simulink model "etrobocon_host"  (R2013b)
settings: Solver=FixedStepDiscrete  StartTime=0.0  StopTime=inf  FixedStep=Ts  RelTol=1e-3
PreLoadFcn:
  | %addpath('C:\Users\ming\Desktop\LEGO_NXT\ETRoboCon2013\data_types\enumerations');
  | Ts = 0.1;
undefined symbols (not defined in the file or in its folder): Green, led0, Stateflow
libraries: embdlinuxlib x11, simulink x6, aerolibanimutils x1
CloseFcn:
  | rmpath('C:\Users\ming\Desktop\LEGO_NXT\ETRoboCon2013\data_types\enumerations');
settings Model: ExtModeTrigDuration=100  Creator=scastro  LastModifiedBy=ming
settings OptimizationCC: OptimizeModelRefInitCode=on  LifeSpan=Inf
settings DebuggingCC: SolverPrmCheckMsg=none
settings HardwareCC: ProdLargestAtomicInteger=Long  ProdLargestAtomicFloat=Double  ProdEndianess=LittleEndian  ProdHWDeviceType=ARM Compatible->ARM Cortex
settings RTWCC: SystemTargetFile=realtime.tlc  GenerateMakefile=off  TemplateMakefile=realtime.tmf  Description=Run on Target Hardware  RTWVerbose=off  ProcessScript=realtime_make_rtw_hook
settings STFCustomTargetCC: TargetLibSuffix=.a  GenerateSampleERTMain=on  ERTCustomFileBanners=on  SupportNonInlinedSFcns=off  SupportVariableSizeSignals=on  MATLABClassNameForMDSCustomization=Simulink.SoftwareTarget.ERTCustomization  GRTInterface=off  SystemTargetFile=realtime.tlc
settings ERTTargetCC: CodeReplacementLibrary=ANSI_C  GenerateSampleERTMain=on  ParMdlRefBuildCompliant=off  CompOptLevelCompliant=off  ConcurrentExecutionCompliant=off  CombineOutputUpdateFcns=off  ERTFirstTimeCompliant=off  SupportContinuousTime=on  SupportVariableSizeSignals=on  ModelStepFunctionPrototypeControlCompliant=off  CPPClassGenCompliant=off  ExtModeMexArgs='192.168.2.6' 0 17725  InlinedParameterPlacement=NonHierarchical  ERTSrcFileBannerTemplate=realtime_code_template.cgt  ERTHdrFileBannerTemplate=realtime_code_template.cgt  ERTDataSrcFileTemplate=realtime_code_template.cgt  ERTDataHdrFileTemplate=realtime_code_template.cgt  ERTCustomFileTemplate=realtime_file_process.tlc

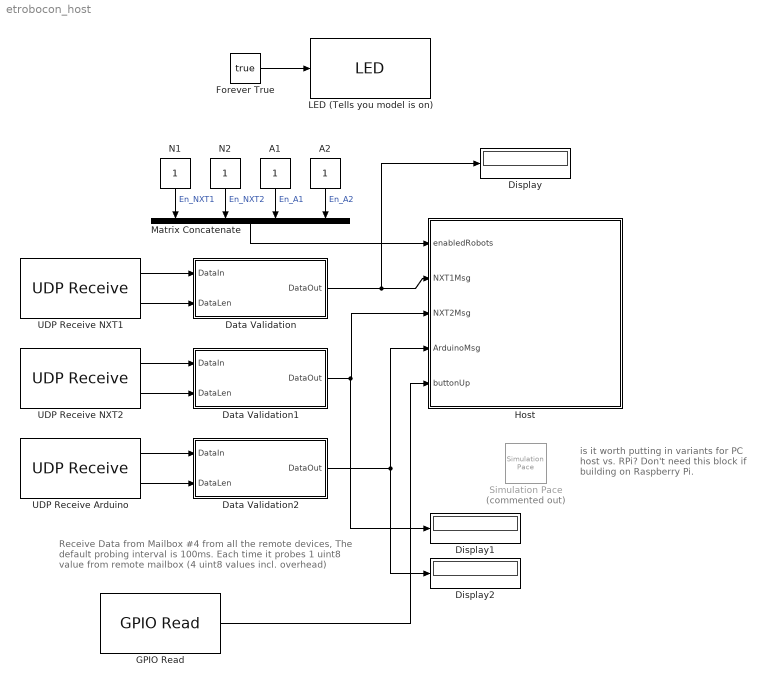
== system etrobocon_host ==
  note: is it worth putting in variants for
      | PC host vs. RPi?
      |
      | Don't need this block if building on
      | Raspberry Pi.
  note: Receive Data from Mailbox #4 from all the remote devices,
      | The default probing interval is 100ms. Each time it probes 1
      | uint8 value from remote mailbox (4 uint8 values incl. overhead)
  A1 : Constant
  A2 : Constant
  Data Validation : Subsystem
  Data Validation1 : Subsystem
  Data Validation2 : Subsystem
  Display : Display
  Display1 : Display
  Display2 : Display
  Forever True : Constant  Value=true  OutDataTypeStr=boolean
  GPIO Read : embdlinuxlib/GPIO Read  board=Model B Rev2  gpio=4  internalResistor=Off  sampleTime=Ts  direction=Input  blockPlatform=Raspberry Pi
  Host : Stateflow chart  TreatAsAtomicUnit=on
  LED (Tells you model is on) : embdlinuxlib/LED  board=Model B Rev2  led=led0 (Green)  blockPlatform=Raspberry Pi
  Matrix Concatenate : Concatenate  NumInputs=4  ConcatenateDimension=2
  N1 : Constant
  N2 : Constant
  Simulation Pace : aerolibanimutils/Simulation Pace  Commented=on  SimulationPace=1  SleepMode=MATLAB Thread  OutputPaceError=off  SampleTime=-1
      settings: AttributesFormatString=%<SimulationPace> sec/sec
  UDP Receive Arduino : embdlinuxlib/UDP Receive  localURL='0.0.0.0'  localPort=35715  remoteURL='0.0.0.0'  remotePort=-1  recvBufferSize=8192  signalDatatype=uint8  dims=4  isVarSize=off  showBlockingTime=off  blockingTime=0  sampletime=Ts  blockPlatform=Raspberry Pi
  "UDP Receive NXT1 " : embdlinuxlib/UDP Receive  localURL='0.0.0.0'  localPort=35713  remoteURL='0.0.0.0'  remotePort=-1  recvBufferSize=8192  signalDatatype=uint8  dims=4  isVarSize=off  showBlockingTime=off  blockingTime=0  sampletime=Ts  blockPlatform=Raspberry Pi
  UDP Receive NXT2 : embdlinuxlib/UDP Receive  localURL='0.0.0.0'  localPort=35714  remoteURL='0.0.0.0'  remotePort=-1  recvBufferSize=8192  signalDatatype=uint8  dims=4  isVarSize=off  showBlockingTime=off  blockingTime=0  sampletime=Ts  blockPlatform=Raspberry Pi
  wires:
  Data Validation/1(DataOut) -> Display/1, Host/2(NXT1Msg)
  N1/1 -> Matrix Concatenate/1  "En_NXT1"
  N2/1 -> Matrix Concatenate/2  "En_NXT2"
  A1/1 -> Matrix Concatenate/3  "En_A1"
  A2/1 -> Matrix Concatenate/4  "En_A2"
  Matrix Concatenate/1 -> Host/1(enabledRobots)
  UDP Receive Arduino/1 -> Data Validation2/1(DataIn)
  UDP Receive Arduino/2 -> Data Validation2/2(DataLen)
  "UDP Receive NXT1 "/2 -> Data Validation/2(DataLen)
  "UDP Receive NXT1 "/1 -> Data Validation/1(DataIn)
  UDP Receive NXT2/2 -> Data Validation1/2(DataLen)
  UDP Receive NXT2/1 -> Data Validation1/1(DataIn)
  Data Validation1/1(DataOut) -> Display1/1, Host/3(NXT2Msg)
  Data Validation2/1(DataOut) -> Host/4(ArduinoMsg), Display2/1
  GPIO Read/1 -> Host/5(buttonUp)
  Forever True/1 -> LED (Tells you model is on)/1

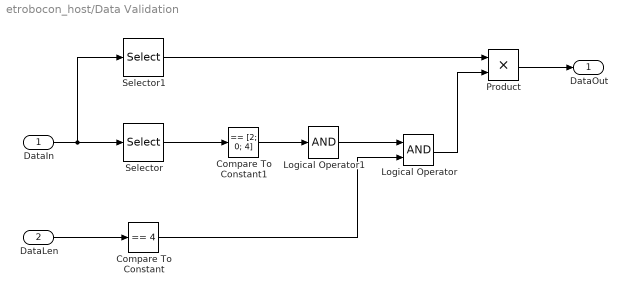
== system etrobocon_host/Data Validation ==
  DataIn : Inport
  DataLen : Inport  Port=2
  Compare To Constant : simulink/Logic and Bit Operations/Compare To Constant  relop===  const=4  OutDataTypeStr=boolean
  Compare To Constant1 : simulink/Logic and Bit Operations/Compare To Constant  relop===  const=[2; 0; 4]  OutDataTypeStr=boolean
  Logical Operator : Logic  AllPortsSameDT=off  OutDataTypeStr=boolean
  Logical Operator1 : Logic  Inputs=1  AllPortsSameDT=off  OutDataTypeStr=boolean
  Product : Product  OutDataTypeStr=uint8
  Selector : Selector  InputPortWidth=4  IndexOptions=Index vector (dialog)  Indices=[1 2 3]  OutputSizes=1
  Selector1 : Selector  InputPortWidth=4  IndexOptions=Index vector (dialog)  Indices=[4]  OutputSizes=1
  DataOut : Outport
  wires:
  Logical Operator/1 -> Product/2
  Compare To Constant/1 -> Logical Operator/2
  Logical Operator1/1 -> Logical Operator/1
  DataIn/1 -> Selector1/1, Selector/1
  DataLen/1 -> Compare To Constant/1
  Selector/1 -> Compare To Constant1/1
  Compare To Constant1/1 -> Logical Operator1/1
  Selector1/1 -> Product/1
  Product/1 -> DataOut/1

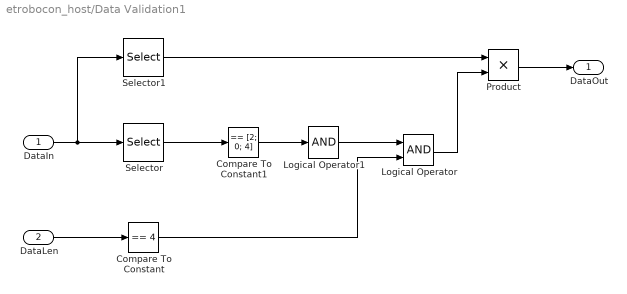
== system etrobocon_host/Data Validation1 ==
  DataIn : Inport
  DataLen : Inport  Port=2
  Compare To Constant : simulink/Logic and Bit Operations/Compare To Constant  relop===  const=4  OutDataTypeStr=boolean
  Compare To Constant1 : simulink/Logic and Bit Operations/Compare To Constant  relop===  const=[2; 0; 4]  OutDataTypeStr=boolean
  Logical Operator : Logic  AllPortsSameDT=off  OutDataTypeStr=boolean
  Logical Operator1 : Logic  Inputs=1  AllPortsSameDT=off  OutDataTypeStr=boolean
  Product : Product  OutDataTypeStr=uint8
  Selector : Selector  InputPortWidth=4  IndexOptions=Index vector (dialog)  Indices=[1 2 3]  OutputSizes=1
  Selector1 : Selector  InputPortWidth=4  IndexOptions=Index vector (dialog)  Indices=[4]  OutputSizes=1
  DataOut : Outport
  wires:
  Product/1 -> DataOut/1
  Selector1/1 -> Product/1
  Compare To Constant1/1 -> Logical Operator1/1
  Selector/1 -> Compare To Constant1/1
  DataLen/1 -> Compare To Constant/1
  DataIn/1 -> Selector/1, Selector1/1
  Logical Operator1/1 -> Logical Operator/1
  Compare To Constant/1 -> Logical Operator/2
  Logical Operator/1 -> Product/2

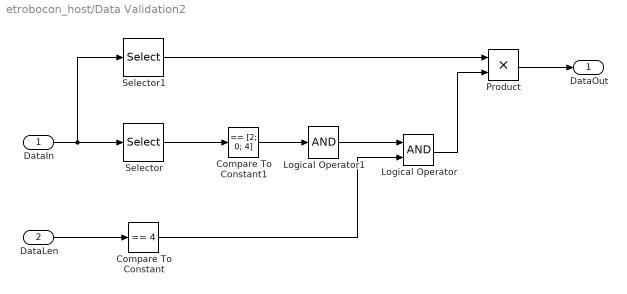
== system etrobocon_host/Data Validation2 ==
  DataIn : Inport
  DataLen : Inport  Port=2
  Compare To Constant : simulink/Logic and Bit Operations/Compare To Constant  relop===  const=4  OutDataTypeStr=boolean
  Compare To Constant1 : simulink/Logic and Bit Operations/Compare To Constant  relop===  const=[2; 0; 4]  OutDataTypeStr=boolean
  Logical Operator : Logic  AllPortsSameDT=off  OutDataTypeStr=boolean
  Logical Operator1 : Logic  Inputs=1  AllPortsSameDT=off  OutDataTypeStr=boolean
  Product : Product  OutDataTypeStr=uint8
  Selector : Selector  InputPortWidth=4  IndexOptions=Index vector (dialog)  Indices=[1 2 3]  OutputSizes=1
  Selector1 : Selector  InputPortWidth=4  IndexOptions=Index vector (dialog)  Indices=[4]  OutputSizes=1
  DataOut : Outport
  wires:
  Logical Operator/1 -> Product/2
  Compare To Constant/1 -> Logical Operator/2
  Logical Operator1/1 -> Logical Operator/1
  DataIn/1 -> Selector1/1, Selector/1
  DataLen/1 -> Compare To Constant/1
  Selector/1 -> Compare To Constant1/1
  Compare To Constant1/1 -> Logical Operator1/1
  Selector1/1 -> Product/1
  Product/1 -> DataOut/1

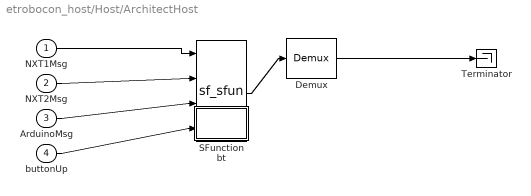
== system etrobocon_host/Host/ArchitectHost ==
  NXT1Msg : Inport
  NXT2Msg : Inport  Port=2
  ArduinoMsg : Inport  Port=3
  buttonUp : Inport  Port=4
  " Demux " : Demux  Outputs=1
  " SFunction " : S-Function  Tag=Stateflow S-Function etrobocon_host 5  FunctionName=sf_sfun  PortCounts=[4 1]  EnableBusSupport=off
  " Terminator " : Terminator
  bt : Stateflow chart  TreatAsAtomicUnit=on
  wires:
  NXT1Msg/1 -> " SFunction "/1
  NXT2Msg/1 -> " SFunction "/2
  ArduinoMsg/1 -> " SFunction "/3
  buttonUp/1 -> " SFunction "/4
  " Demux "/1 -> " Terminator "/1
  " SFunction "/1 -> " Demux "/1

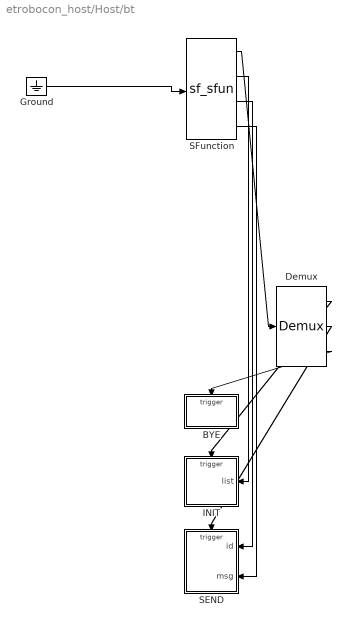
== system etrobocon_host/Host/bt ==
  " Demux " : Demux  Outputs=3
  " Ground " : Ground
  " SFunction " : S-Function  Tag=Stateflow S-Function etrobocon_host 2  FunctionName=sf_sfun  PortCounts=[1 4]  EnableBusSupport=off
  BYE : Subsystem
      settings: UndoDeleteFcn=Stateflow.SLINSF.SimulinkMan.restorePreDeleteFcn  PreDeleteFcn=Stateflow.SLINSF.SimulinkMan.removePreDeleteFcn
  INIT : Subsystem
      settings: UndoDeleteFcn=Stateflow.SLINSF.SimulinkMan.restorePreDeleteFcn  PreDeleteFcn=Stateflow.SLINSF.SimulinkMan.removePreDeleteFcn
  SEND : Subsystem
      settings: UndoDeleteFcn=Stateflow.SLINSF.SimulinkMan.restorePreDeleteFcn  PreDeleteFcn=Stateflow.SLINSF.SimulinkMan.removePreDeleteFcn
  wires:
  " SFunction "/2 -> INIT/1(list)
  " Demux "/1 -> INIT/Trigger
  " SFunction "/3 -> SEND/1(id)
  " SFunction "/4 -> SEND/2(msg)
  " Demux "/2 -> SEND/Trigger
  " Demux "/3 -> BYE/Trigger
  " Ground "/1 -> " SFunction "/1
  " SFunction "/1 -> " Demux "/1

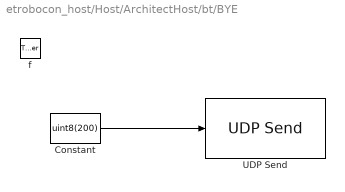
== system etrobocon_host/Host/ArchitectHost/bt/BYE ==
  f : TriggerPort  TriggerType=function-call
      settings: CopyFcn=Stateflow.SLINSF.SimulinkMan.removeBlockPreDeleteFcn  PreDeleteFcn=Stateflow.SLINSF.SimulinkMan.unsafePredeleteFcn
  Constant : Constant  Value=uint8(200)  VectorParams1D=off
      settings: SamplingMode=Frame based
  UDP Send : embdlinuxlib/UDP Send  remoteURL='127.0.0.1'  remotePort=35712  localURL='255.255.255.255'  localPortSource=Automatically determine  localPort=-1  sampletime=-1  blockPlatform=Raspberry Pi  separateLengthPort=0
  wires:
  Constant/1 -> UDP Send/1

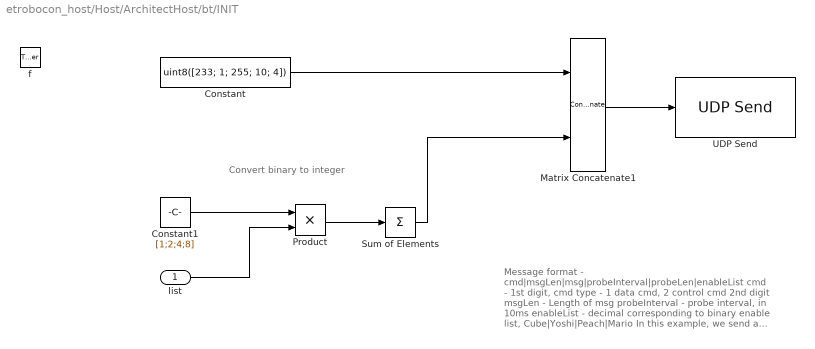
== system etrobocon_host/Host/ArchitectHost/bt/INIT ==
  note: Message format -
      | cmd|msgLen|msg|probeInterval|probeLen|enableList
      | cmd - 1st digit, cmd type - 1 data cmd, 2 control cmd
      | 2nd digit
      | msgLen - Length of msg
      | probeInterval - probe interval, in 10ms
      | enableList - decimal corresponding to binary enable list,
      | Cube|Yoshi|Peach|Mario
      | In this example, we send a unint8 255
  note: Convert binary to integer
  list : Inport  OutDataTypeStr=double  PortDimensions=4
  f : TriggerPort  TriggerType=function-call
      settings: CopyFcn=Stateflow.SLINSF.SimulinkMan.removeBlockPreDeleteFcn  PreDeleteFcn=Stateflow.SLINSF.SimulinkMan.unsafePredeleteFcn
  Constant : Constant  Value=uint8([233; 1; 255; 10; 4])  VectorParams1D=off
      settings: SamplingMode=Frame based
  Constant1 : Constant  Value=[1;2;4;8]
  Matrix Concatenate1 : Concatenate  Mode=Multidimensional array
  Product : Product
  Sum of Elements : Sum  Inputs=+  AccumDataTypeStr=uint8  OutDataTypeStr=uint8
  UDP Send : embdlinuxlib/UDP Send  remoteURL='127.0.0.1'  remotePort=35712  localURL='255.255.255.255'  localPortSource=Automatically determine  localPort=-1  sampletime=-1  blockPlatform=Raspberry Pi  separateLengthPort=0
  wires:
  Sum of Elements/1 -> Matrix Concatenate1/2
  Constant/1 -> Matrix Concatenate1/1
  Matrix Concatenate1/1 -> UDP Send/1
  Product/1 -> Sum of Elements/1
  Constant1/1 -> Product/1
  list/1 -> Product/2

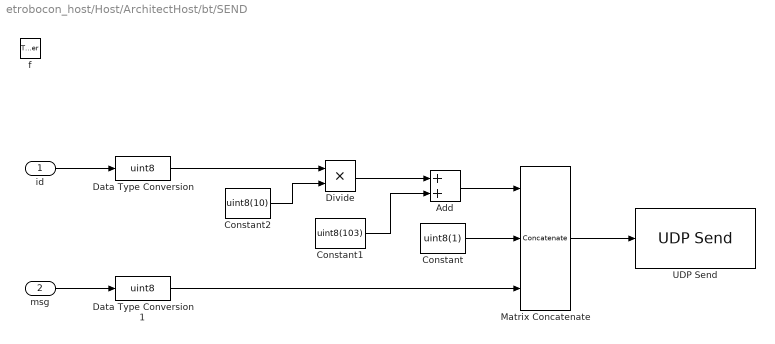
== system etrobocon_host/Host/ArchitectHost/bt/SEND ==
  id : Inport  OutDataTypeStr=Enum: RobotID  PortDimensions=1
  msg : Inport  Port=2  OutDataTypeStr=Enum: StatusID  PortDimensions=1
  f : TriggerPort  TriggerType=function-call
      settings: CopyFcn=Stateflow.SLINSF.SimulinkMan.removeBlockPreDeleteFcn  PreDeleteFcn=Stateflow.SLINSF.SimulinkMan.unsafePredeleteFcn
  Add : Sum
  Constant : Constant  Value=uint8(1)  VectorParams1D=off
  Constant1 : Constant  Value=uint8(103)  VectorParams1D=off
  Constant2 : Constant  Value=uint8(10)  VectorParams1D=off
  Data Type Conversion : DataTypeConversion  OutDataTypeStr=uint8
  Data Type Conversion1 : DataTypeConversion  OutDataTypeStr=uint8
  Divide : Product  Inputs=**  OutDataTypeStr=uint8
  Matrix Concatenate : Concatenate  NumInputs=3  Mode=Multidimensional array
  UDP Send : embdlinuxlib/UDP Send  remoteURL='127.0.0.1'  remotePort=35712  localURL='255.255.255.255'  localPortSource=Automatically determine  localPort=-1  sampletime=-1  blockPlatform=Raspberry Pi  separateLengthPort=0
  wires:
  Data Type Conversion1/1 -> Matrix Concatenate/3
  Data Type Conversion/1 -> Divide/1
  Add/1 -> Matrix Concatenate/1
  Divide/1 -> Add/1
  id/1 -> Data Type Conversion/1
  Constant1/1 -> Add/2
  Constant2/1 -> Divide/2
  Constant/1 -> Matrix Concatenate/2
  msg/1 -> Data Type Conversion1/1
  Matrix Concatenate/1 -> UDP Send/1

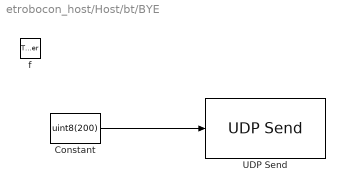
== system etrobocon_host/Host/bt/BYE ==
  f : TriggerPort  TriggerType=function-call
      settings: CopyFcn=Stateflow.SLINSF.SimulinkMan.removeBlockPreDeleteFcn  PreDeleteFcn=Stateflow.SLINSF.SimulinkMan.unsafePredeleteFcn
  Constant : Constant  Value=uint8(200)  VectorParams1D=off
      settings: SamplingMode=Frame based
  UDP Send : embdlinuxlib/UDP Send  remoteURL='127.0.0.1'  remotePort=35712  localURL='255.255.255.255'  localPortSource=Automatically determine  localPort=-1  sampletime=-1  blockPlatform=Raspberry Pi  separateLengthPort=0
  wires:
  Constant/1 -> UDP Send/1

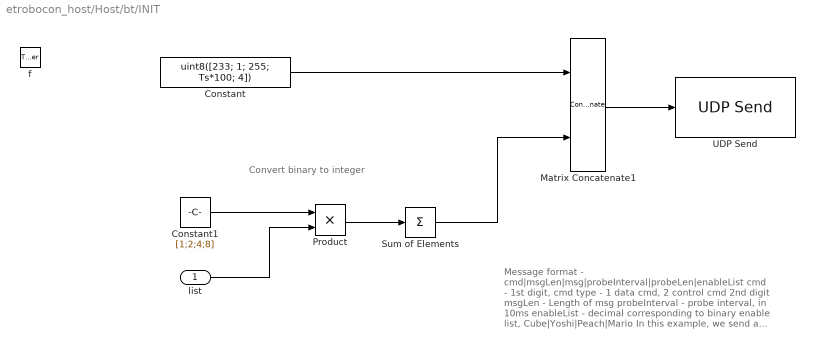
== system etrobocon_host/Host/bt/INIT ==
  note: Message format -
      | cmd|msgLen|msg|probeInterval|probeLen|enableList
      | cmd - 1st digit, cmd type - 1 data cmd, 2 control cmd
      | 2nd digit
      | msgLen - Length of msg
      | probeInterval - probe interval, in 10ms
      | enableList - decimal corresponding to binary enable list,
      | Cube|Yoshi|Peach|Mario
      | In this example, we send a unint8 255
  note: Convert binary to integer
  list : Inport  OutDataTypeStr=double  PortDimensions=4
  f : TriggerPort  TriggerType=function-call
      settings: CopyFcn=Stateflow.SLINSF.SimulinkMan.removeBlockPreDeleteFcn  PreDeleteFcn=Stateflow.SLINSF.SimulinkMan.unsafePredeleteFcn
  Constant : Constant  Value=uint8([233; 1; 255; Ts*100; 4])  VectorParams1D=off
      settings: SamplingMode=Frame based
  Constant1 : Constant  Value=[1;2;4;8]
  Matrix Concatenate1 : Concatenate  Mode=Multidimensional array
  Product : Product
  Sum of Elements : Sum  Inputs=+  AccumDataTypeStr=uint8  OutDataTypeStr=uint8
  UDP Send : embdlinuxlib/UDP Send  remoteURL='127.0.0.1'  remotePort=35712  localURL='255.255.255.255'  localPortSource=Automatically determine  localPort=-1  sampletime=-1  blockPlatform=Raspberry Pi  separateLengthPort=0
  wires:
  list/1 -> Product/2
  Constant1/1 -> Product/1
  Product/1 -> Sum of Elements/1
  Sum of Elements/1 -> Matrix Concatenate1/2
  Constant/1 -> Matrix Concatenate1/1
  Matrix Concatenate1/1 -> UDP Send/1

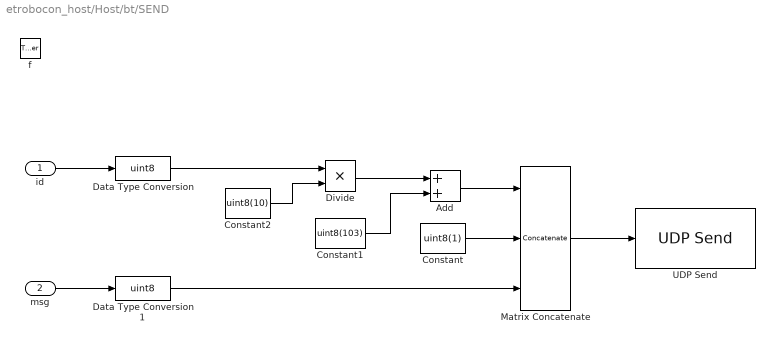
== system etrobocon_host/Host/bt/SEND ==
  id : Inport  OutDataTypeStr=Enum: RobotID  PortDimensions=1
  msg : Inport  Port=2  OutDataTypeStr=Enum: StatusID  PortDimensions=1
  f : TriggerPort  TriggerType=function-call
      settings: CopyFcn=Stateflow.SLINSF.SimulinkMan.removeBlockPreDeleteFcn  PreDeleteFcn=Stateflow.SLINSF.SimulinkMan.unsafePredeleteFcn
  Add : Sum
  Constant : Constant  Value=uint8(1)  VectorParams1D=off
  Constant1 : Constant  Value=uint8(103)  VectorParams1D=off
  Constant2 : Constant  Value=uint8(10)  VectorParams1D=off
  Data Type Conversion : DataTypeConversion  OutDataTypeStr=uint8
  Data Type Conversion1 : DataTypeConversion  OutDataTypeStr=uint8
  Divide : Product  Inputs=**  OutDataTypeStr=uint8
  Matrix Concatenate : Concatenate  NumInputs=3  Mode=Multidimensional array
  UDP Send : embdlinuxlib/UDP Send  remoteURL='127.0.0.1'  remotePort=35712  localURL='255.255.255.255'  localPortSource=Automatically determine  localPort=-1  sampletime=-1  blockPlatform=Raspberry Pi  separateLengthPort=0
  wires:
  Data Type Conversion1/1 -> Matrix Concatenate/3
  Data Type Conversion/1 -> Divide/1
  Add/1 -> Matrix Concatenate/1
  Divide/1 -> Add/1
  id/1 -> Data Type Conversion/1
  Constant1/1 -> Add/2
  Constant2/1 -> Divide/2
  Constant/1 -> Matrix Concatenate/2
  msg/1 -> Data Type Conversion1/1
  Matrix Concatenate/1 -> UDP Send/1

== stateflow chart etrobocon_host/Host/bt ==
  state INIT(list) [function]
  state SEND(id,msg) [function]
  state BYE [function]
  data: list function_input double size=4; id function_input Enum: RobotID size=1; msg function_input Enum: StatusID size=1

== stateflow chart etrobocon_host/Host ==
  settings: updateMethod=DISCRETE  sampleTime=Ts
  state Init_wait
    en:
  note: Bluetooth Functions here
      | bt.INIT(list)
      | bt.SEND(id,msg)
      | bt.BYE()
  state Initialize
    en: bt.INIT(enabledRobots);
  state bt [group]
  state ArchitectHost
  state Terminate
    en: bt.BYE;
  (default) -> Init_wait
  Init_wait -> Initialize : [hasChangedFrom(buttonUp,0)]
  Terminate -> Initialize : [hasChangedFrom(buttonUp,0)]
  Initialize -> ArchitectHost
  ArchitectHost -> Terminate : % Broadcast this from
      | % your atomic subchart
      | % to terminate comm
      | [done]
  data: enabledRobots input; NXT1Msg input; NXT2Msg input; ArduinoMsg input; done local boolean size=1; buttonUp input

== stateflow chart etrobocon_host/Host/ArchitectHost ==
  state bt [group]
  state NormalOperation
    state TellCubeToHeart
      en:
      bt.SEND(RobotID.LEDCUBE, StatusID.HEART);
    state Wait
    state TellNXT2ToStand
      en:
      bt.SEND(RobotID.NXT2, StatusID.NXT2_STAND);
    state TellCubeToStar
      en:
      bt.SEND(RobotID.LEDCUBE, StatusID.STAR);
    state TellNXT2ToStartMoving
      en:
      bt.SEND(RobotID.NXT2, StatusID.NXT2_START);
    state TellNXT1ToGoBack
      en:
      bt.SEND(RobotID.NXT1, StatusID.NXT1_GO_BACK);
    state TellMarioToLeaveRamp
      en:
      bt.SEND(RobotID.NXT1, StatusID.NXT1_GO_DOWN_RAMP);
    state TellNXT2ToFollow
      en:
      bt.SEND(RobotID.NXT2, StatusID.NXT2_FOLLOW);
    state TellNXT1ToSpeedUp
      en:
      bt.SEND(RobotID.NXT1, StatusID.NXT1_SPEED_UP);
    state TellNXT2ToWait
      en:
      bt.SEND(RobotID.NXT2, StatusID.NXT2_WAIT);
      bt.SEND(RobotID.LEDCUBE, StatusID.FIREWORKS);
    state TellNXT2ToGetOffSeesaw
      en:
      bt.SEND(RobotID.NXT2, StatusID.NXT2_LEAVE);
    state TellNXT1ToPark
      en:
      bt.SEND(RobotID.NXT1, StatusID.NXT1_PARK);
    (default) -> Wait
    TellMarioToLeaveRamp -> TellCubeToHeart : [isequal(NXT1Msg,StatusID.NXT1_OFF_RAMP)]
    TellCubeToHeart -> TellNXT2ToStand : [isequal(NXT1Msg,StatusID.NXT1_ON_SEESAW)]
    Wait -> TellCubeToStar : [isequal(NXT1Msg,StatusID.NXT1_AT_STAGE)]
    TellNXT2ToStand -> TellNXT2ToStartMoving : [isequal(NXT1Msg,StatusID.NXT1_WAITING)]
    TellCubeToStar -> TellMarioToLeaveRamp : [isequal(ArduinoMsg,StatusID.ROVER_SENSED_RAMP)]
    TellNXT2ToStartMoving -> TellNXT1ToGoBack : [isequal(NXT2Msg,StatusID.NXT2_ON_SEESAW)]
    TellNXT1ToGoBack -> TellNXT2ToFollow : [isequal(NXT1Msg,StatusID.NXT1_ON_PIVOT)]
    TellNXT2ToFollow -> TellNXT1ToSpeedUp : [isequal(NXT2Msg,StatusID.NXT2_IN_HURRY)]
    TellNXT1ToSpeedUp -> TellNXT2ToWait : [isequal(NXT1Msg,StatusID.NXT1_OFF_SEESAW)]
    TellNXT2ToWait -> TellNXT2ToGetOffSeesaw : [isequal(NXT1Msg,StatusID.NXT1_TURNED)]
    TellNXT2ToGetOffSeesaw -> TellNXT1ToPark : [isequal(NXT2Msg,StatusID.NXT2_READY_TO_PARK)]
  state Off
    en:
    done = true;
  (default) -> NormalOperation : {done=false;}
  NormalOperation -> Off : [hasChangedFrom(buttonUp,0)]
  data: NXT1Msg input; NXT2Msg input; ArduinoMsg input; done data_store_memory; buttonUp input boolean

== stateflow chart etrobocon_host/Host/ArchitectHost/bt ==
  state INIT(list) [function]
  state SEND(id,msg) [function]
  state BYE [function]
  data: list function_input double size=4; id function_input Enum: RobotID size=1; msg function_input Enum: StatusID size=1
